simulink model "drone_problem"  (R2022b)
settings: Solver=VariableStepAuto  StartTime=0.0  StopTime=10.0  RelTol=1e-3
values from neighbouring files (symbols this model uses):
  F_x_g = 0.0    (= 0)    [params.m]
  F_y_g = 0.0    (= 0)    [params.m]
  g = 9.8    [params.m]
  kf = 0.005022    [params.m]
  m = 0.034    [params.m]
settings Model: Creator=depressedcoder  LastModifiedBy=depressedcoder

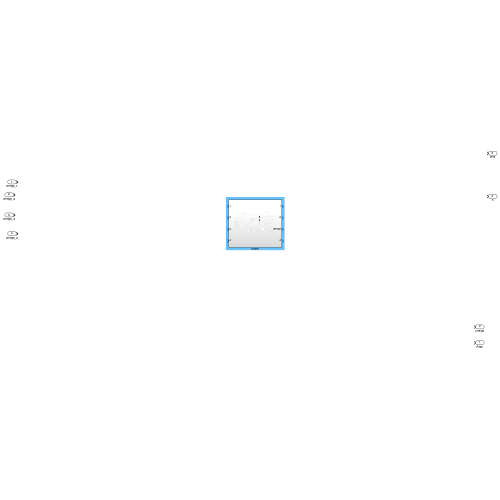
[thumbnail: Simulink's stored preview of the top-level diagram]
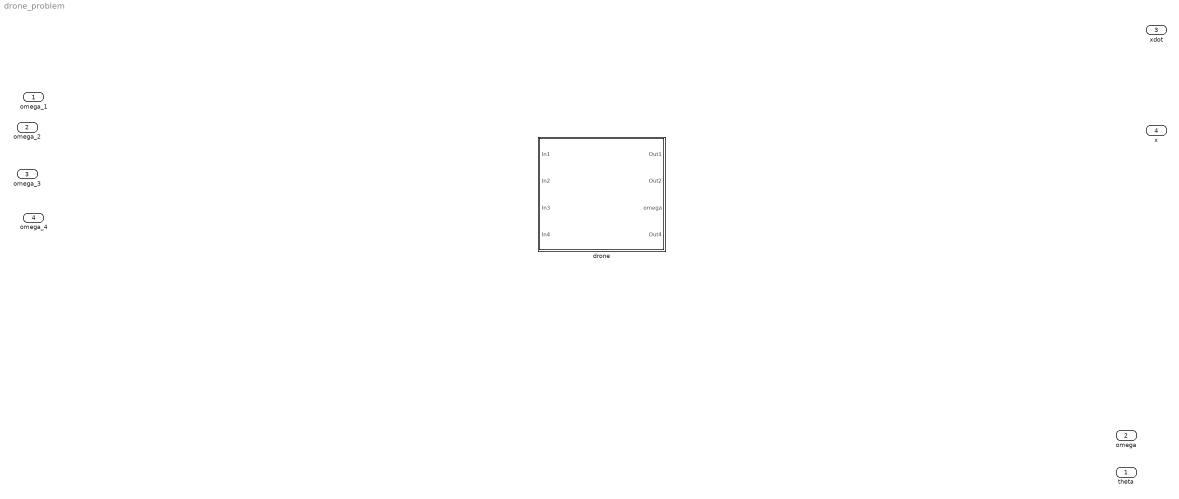
== system drone_problem ==
  omega_1 : Inport
  omega_2 : Inport  Port=2
  omega_3 : Inport  Port=3
  omega_4 : Inport  Port=4
  drone : Subsystem
  theta : Outport
  omega : Outport  Port=2
  xdot : Outport  Port=3
  x : Outport  Port=4

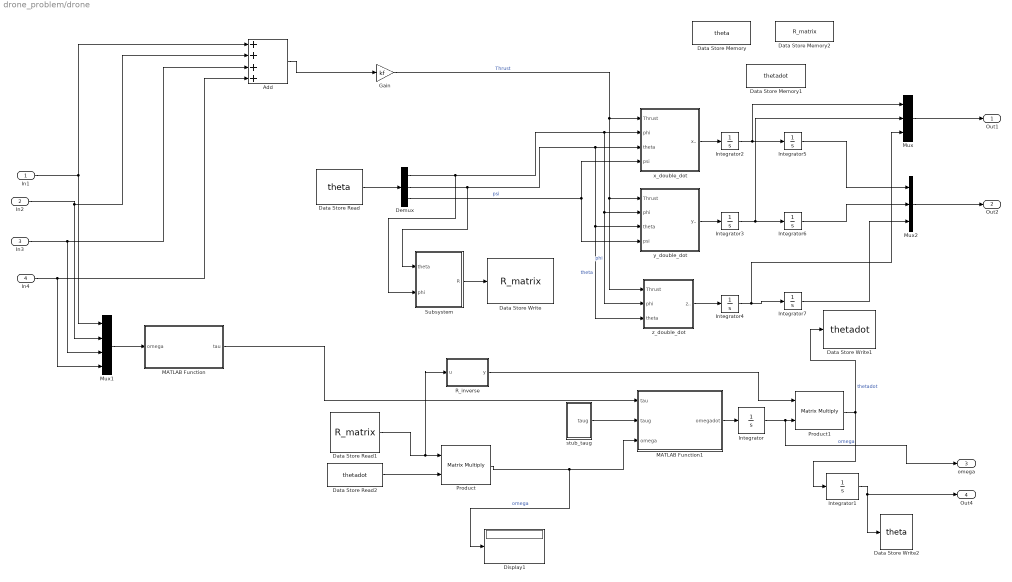
== system drone_problem/drone ==
  In1 : Inport
  In2 : Inport  Port=2
  In3 : Inport  Port=3
  In4 : Inport  Port=4
  Add : Sum  Inputs=++++
  Data Store Memory : DataStoreMemory  DataStoreName=theta  WriteAfterWriteMsg=warning  InitialValue=[0 ; 0 ; 0]  ShowAdditionalParam=off
  Data Store Memory1 : DataStoreMemory  DataStoreName=thetadot  WriteAfterWriteMsg=warning  InitialValue=|  ShowAdditionalParam=off
      | [1.4430 ; 0.4620 ; -1.4048
      | ]
  Data Store Memory2 : DataStoreMemory  DataStoreName=R_matrix  WriteAfterWriteMsg=warning  InitialValue=[ 1 0 0 ; 0 1 0 ; 0 0 1 ]  ShowAdditionalParam=off
  Data Store Read : DataStoreRead  DataStoreName=theta  IndexOptions=Index vector (dialog)  Indices=1  OutputSizes=1
  Data Store Read1 : DataStoreRead  DataStoreName=R_matrix  IndexOptions=Index vector (dialog)  Indices=1  OutputSizes=1
  Data Store Read2 : DataStoreRead  DataStoreName=thetadot  IndexOptions=Index vector (dialog)  Indices=1  OutputSizes=1
  Data Store Write : DataStoreWrite  DataStoreName=R_matrix  IndexOptions=Index vector (dialog)  Indices=1  OutputSizes=1
  Data Store Write1 : DataStoreWrite  DataStoreName=thetadot  IndexOptions=Index vector (dialog)  Indices=1  OutputSizes=1
  Data Store Write2 : DataStoreWrite  DataStoreName=theta  IndexOptions=Index vector (dialog)  Indices=1  OutputSizes=1
  Demux : Demux  Outputs=3
  Display1 : Display
  Gain : Gain  Gain=kf
  Integrator{,1..7} (8 alike) : Integrator
  MATLAB Function : MATLAB Function  TreatAsAtomicUnit=on
  MATLAB Function1 : MATLAB Function  TreatAsAtomicUnit=on
  Mux : Mux  Inputs=3
  Mux1 : Mux
  Mux2 : Mux  Inputs=3
  Product : Product  Multiplication=Matrix(*)
  Product1 : Product  Multiplication=Matrix(*)
  R_inverse : MATLAB Function  TreatAsAtomicUnit=on
  Subsystem : Subsystem
  stub_taug : Subsystem
  x_double_dot : Subsystem
  y_double_dot : Subsystem
  z_double_dot : Subsystem
  Out1 : Outport
  Out2 : Outport  Port=2
  omega : Outport  Port=3
  Out4 : Outport  Port=4
  wires:
  MATLAB Function1/1(omegadot) -> Integrator/1
  Integrator6/1 -> Mux2/2
  Integrator/1 -> omega/1, Product1/2  "omega"
  MATLAB Function/1(tau) -> MATLAB Function1/1(tau)
  Mux1/1 -> MATLAB Function/1(omega)
  In2/1 -> Mux1/2, Add/2
  Add/1 -> Gain/1
  z_double_dot/1(z..) -> Integrator4/1
  Mux/1 -> Out1/1
  Subsystem/1(R) -> Data Store Write/1
  Mux2/1 -> Out2/1
  stub_taug/1(taug) -> MATLAB Function1/2(taug)
  y_double_dot/1(y..) -> Integrator3/1
  R_inverse/1(y) -> Product1/1
  Product1/1 -> Integrator1/1, Data Store Write1/1  "thetadot"
  In4/1 -> Mux1/4, Add/4
  Integrator3/1 -> Mux/2, Integrator6/1
  Demux/3 -> x_double_dot/4(psi), y_double_dot/4(psi)  "psi"
  Integrator1/1 -> Out4/1, Data Store Write2/1
  In1/1 -> Mux1/1, Add/1
  Data Store Read2/1 -> Product/2
  Data Store Read1/1 -> R_inverse/1(u), Product/1
  Integrator5/1 -> Mux2/1
  Demux/1 -> Subsystem/2(phi), z_double_dot/2(phi), y_double_dot/2(phi), x_double_dot/2(phi)  "phi"
  Product/1 -> MATLAB Function1/3(omega), Display1/1  "omega"
  Integrator7/1 -> Mux2/3
  Integrator2/1 -> Mux/1, Integrator5/1
  Demux/2 -> Subsystem/1(theta), z_double_dot/3(theta), y_double_dot/3(theta), x_double_dot/3(theta)  "theta"
  x_double_dot/1(x..) -> Integrator2/1
  In3/1 -> Mux1/3, Add/3
  Integrator4/1 -> Mux/3, Integrator7/1
  Data Store Read/1 -> Demux/1
  Gain/1 -> z_double_dot/1(Thrust), y_double_dot/1(Thrust), x_double_dot/1(Thrust)  "Thrust"

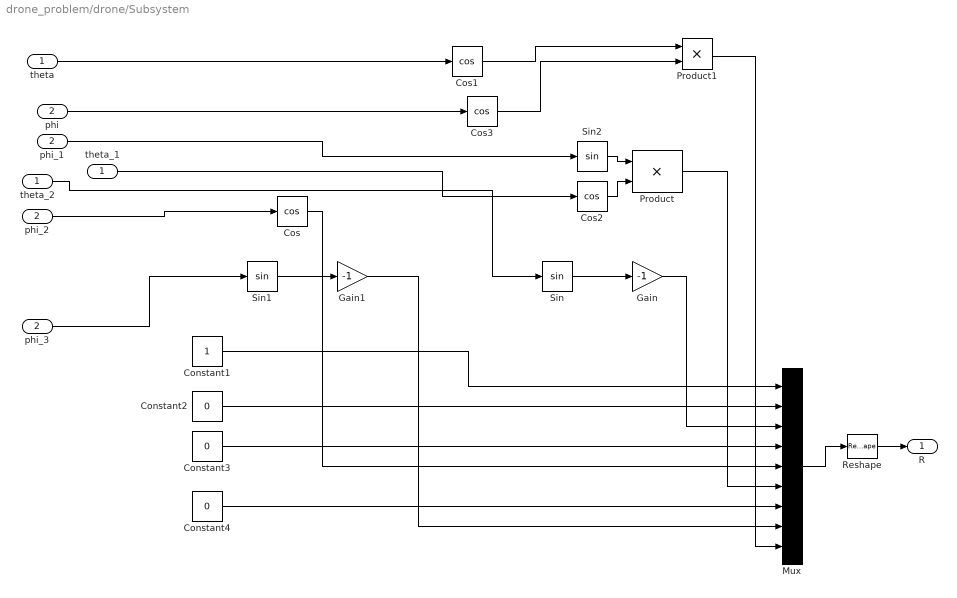
== system drone_problem/drone/Subsystem ==
  theta : Inport
  phi : Inport  Port=2
  Constant1 : Constant
  Constant2 : Constant  Value=0
  Constant3 : Constant  Value=0
  Constant4 : Constant  Value=0
  Cos{,1..3} (4 alike) : Trigonometry  Operator=cos
  Gain : Gain  Gain=-1
  Gain1 : Gain  Gain=-1
  Mux : Mux  Inputs=9
  Product : Product
  Product1 : Product
  Reshape : Reshape  OutputDimensionality=Customize  OutputDimensions=[3,3]
  Sin : Trigonometry
  Sin1 : Trigonometry
  Sin2 : Trigonometry
  phi_1 : InportShadow  Port=2
  phi_2 : InportShadow  Port=2
  phi_3 : InportShadow  Port=2
  theta_1 : InportShadow
  theta_2 : InportShadow
  R : Outport
  wires:
  theta_2/1 -> Sin/1
  Product1/1 -> Mux/9
  Reshape/1 -> R/1
  Mux/1 -> Reshape/1
  Constant1/1 -> Mux/1
  phi_1/1 -> Sin2/1
  phi_3/1 -> Sin1/1
  Cos2/1 -> Product/2
  Product/1 -> Mux/6
  Sin2/1 -> Product/1
  Constant2/1 -> Mux/2
  Sin/1 -> Gain/1
  Constant4/1 -> Mux/7
  Cos3/1 -> Product1/2
  phi/1 -> Cos3/1
  theta_1/1 -> Cos2/1
  theta/1 -> Cos1/1
  Gain/1 -> Mux/3
  Sin1/1 -> Gain1/1
  phi_2/1 -> Cos/1
  Constant3/1 -> Mux/4
  Gain1/1 -> Mux/8
  Cos1/1 -> Product1/1
  Cos/1 -> Mux/5

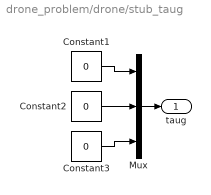
== system drone_problem/drone/stub_taug ==
  Constant1 : Constant  Value=0
  Constant2 : Constant  Value=0
  Constant3 : Constant  Value=0
  Mux : Mux  Inputs=3
  taug : Outport
  wires:
  Constant3/1 -> Mux/3
  Constant1/1 -> Mux/1
  Mux/1 -> taug/1
  Constant2/1 -> Mux/2

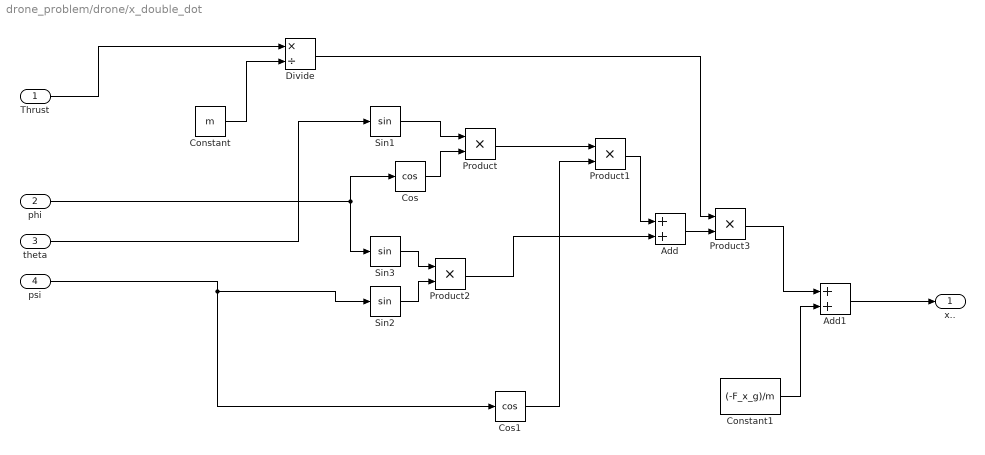
== system drone_problem/drone/x_double_dot ==
  Thrust : Inport
  phi : Inport  Port=2
  theta : Inport  Port=3
  psi : Inport  Port=4
  Add : Sum
  Add1 : Sum
  Constant : Constant  Value=m
  Constant1 : Constant  Value=(-F_x_g)/m
  Cos : Trigonometry  Operator=cos
  Cos1 : Trigonometry  Operator=cos
  Divide : Product  Inputs=*/
  Product{,1..3} (4 alike) : Product
  Sin1 : Trigonometry
  Sin2 : Trigonometry
  Sin3 : Trigonometry
  x.. : Outport
  wires:
  Add1/1 -> x../1
  Product2/1 -> Add/2
  Cos1/1 -> Product1/2
  Product1/1 -> Add/1
  Sin1/1 -> Product/1
  Divide/1 -> Product3/1
  Product3/1 -> Add1/1
  theta/1 -> Sin1/1
  Add/1 -> Product3/2
  Sin2/1 -> Product2/2
  Sin3/1 -> Product2/1
  Thrust/1 -> Divide/1
  Product/1 -> Product1/1
  Cos/1 -> Product/2
  phi/1 -> Cos/1, Sin3/1
  psi/1 -> Cos1/1, Sin2/1
  Constant/1 -> Divide/2
  Constant1/1 -> Add1/2

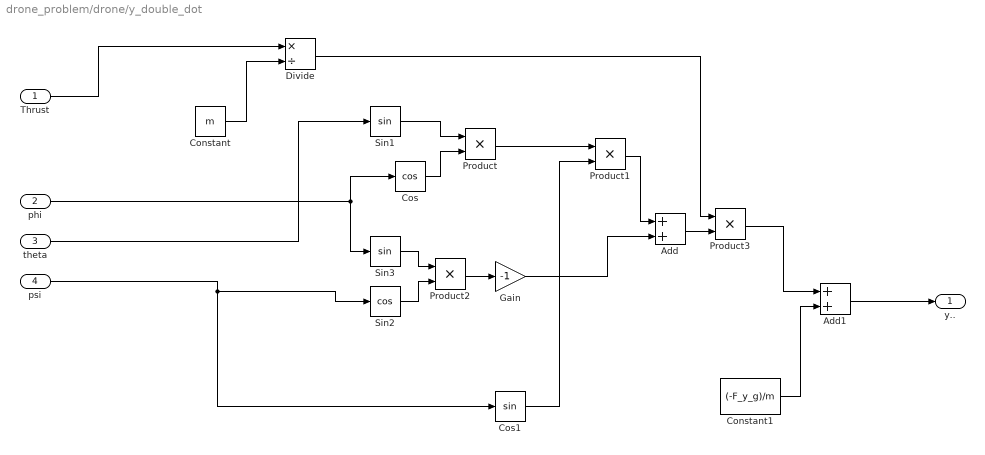
== system drone_problem/drone/y_double_dot ==
  Thrust : Inport
  phi : Inport  Port=2
  theta : Inport  Port=3
  psi : Inport  Port=4
  Add : Sum
  Add1 : Sum
  Constant : Constant  Value=m
  Constant1 : Constant  Value=(-F_y_g)/m
  Cos : Trigonometry  Operator=cos
  Cos1 : Trigonometry
  Divide : Product  Inputs=*/
  Gain : Gain  Gain=-1
  Product{,1..3} (4 alike) : Product
  Sin1 : Trigonometry
  Sin2 : Trigonometry  Operator=cos
  Sin3 : Trigonometry
  y.. : Outport
  wires:
  Constant1/1 -> Add1/2
  Constant/1 -> Divide/2
  psi/1 -> Sin2/1, Cos1/1
  phi/1 -> Sin3/1, Cos/1
  Cos/1 -> Product/2
  Product/1 -> Product1/1
  Thrust/1 -> Divide/1
  Sin3/1 -> Product2/1
  Sin2/1 -> Product2/2
  Add/1 -> Product3/2
  theta/1 -> Sin1/1
  Product3/1 -> Add1/1
  Divide/1 -> Product3/1
  Sin1/1 -> Product/1
  Product1/1 -> Add/1
  Cos1/1 -> Product1/2
  Add1/1 -> y../1
  Product2/1 -> Gain/1
  Gain/1 -> Add/2

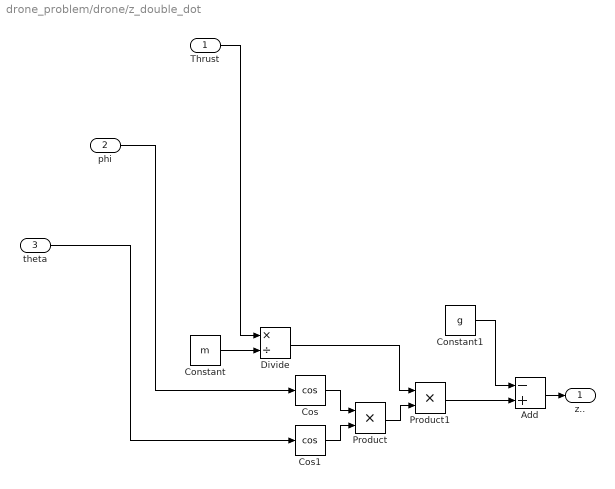
== system drone_problem/drone/z_double_dot ==
  Thrust : Inport
  phi : Inport  Port=2
  theta : Inport  Port=3
  Add : Sum  Inputs=-+
  Constant : Constant  Value=m
  Constant1 : Constant  Value=g
  Cos : Trigonometry  Operator=cos
  Cos1 : Trigonometry  Operator=cos
  Divide : Product  Inputs=*/
  Product : Product
  Product1 : Product
  z.. : Outport
  wires:
  theta/1 -> Cos1/1
  Cos/1 -> Product/1
  Divide/1 -> Product1/1
  Product/1 -> Product1/2
  Constant1/1 -> Add/1
  Add/1 -> z../1
  Thrust/1 -> Divide/1
  Cos1/1 -> Product/2
  Constant/1 -> Divide/2
  phi/1 -> Cos/1
  Product1/1 -> Add/2

== matlab function drone_problem/drone/R_inverse ==
  data: u input; y output
function y = fcn(u)

y = inv(u);

== matlab function drone_problem/drone/MATLAB Function ==
  data: omega input; tau output
function tau = fcn(omega)
kf = 0.005022;
km = 1.858*10^-5;
L = 0.032;
mma = [ 0 kf*L 0 -kf*L ; -kf*L 0 kf*L 0 ; km -km km -km];
tau = mma*omega;

== matlab function drone_problem/drone/MATLAB Function1 ==
  data: tau input; taug input; omegadot output; omega input
function omegadot = fcn(tau,taug,omega)
I = [2.3951*10^-5 0 0 ; 0 2.3951*10^-5 0 ; 0 0 3.2347*10^-5];
output = inv(I)*((tau-taug) - cross(omega,I*omega));
omegadot = output;
